simulink library "MinSegLibrary_M2V3"  (R2015a)
settings: Solver=ode45  StartTime=0.0  StopTime=10.0  RelTol=1e-3
libraries: arduinolib x4
settings Model: Creator=hurstj  LastModifiedBy=008399924
settings DebuggingCC: UnderspecifiedInitializationDetection=Classic  MergeDetectMultiDrivingBlocksExec=none  SolverPrmCheckMsg=warning  StateNameClashWarn=warning

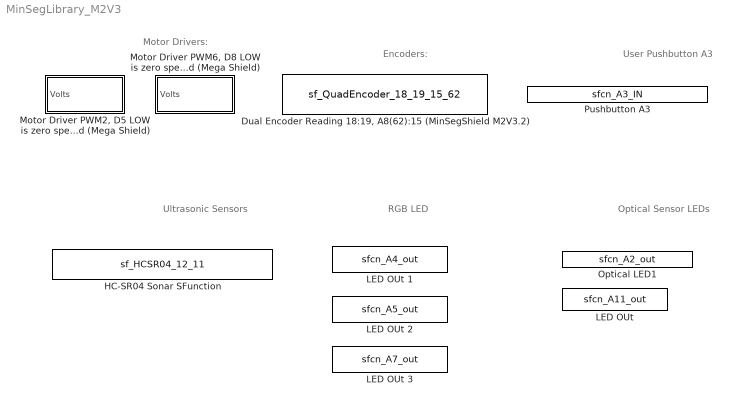
== system MinSegLibrary_M2V3 ==
  note: Motor Drivers:
  note: Ultrasonic Sensors
  note: Encoders:
  note: RGB LED
  note: User Pushbutton A3
  note: Optical Sensor LEDs
  "Dual Encoder Reading 18:19, A8(62):15 (MinSegShield M2V3.2) " : S-Function  InitFcn=try, set_param(gcb,'FunctionName','sf_QuadEncoder_18_19_15_62'), end  FunctionName=sf_QuadEncoder_18_19_15_62  Parameters=uint8([0 1]),uint8([18 62]),uint8([19 15])  SFunctionModules=sf_QuadEncoder_18_19_15_62_wrapper  mask(S-Function Builder){}
      mask init:
      | val = [[.9  0.75 0.75 1 1 .9 .9 1]',[1 1 0.75 0.75 .9 .9 1 .9]'];try , sys = get_param(gcb,'SfunBuilderFcnName');if isempty(sys), sys = get_param(gcb,'FunctionName'); end,catch, sys = get_param(gcb,'FunctionName'); end
      settings: CopyFcn=set_param(gcbh,'LinkStatus','none')  PreSaveFcn=try, set_param(gcb,'FunctionName','sf_QuadEncoder_18_19_15_62'), end  OpenFcn=sfunctionwizard(gcbh)
      mask Display: plot(val(:,1),val(:,2)),disp(sys), port_label('output',1,'pos1'), port_label('output',2,'pos2')
  HC-SR04 Sonar SFunction : S-Function  InitFcn=try, set_param(gcb,'FunctionName','sf_HCSR04_12_11'), end  FunctionName=sf_HCSR04_12_11  SFunctionModules=sf_HCSR04_12_11_wrapper  mask(S-Function Builder){}
      mask help: Simulink:masks:SFunctionBuilder_MD
      mask init: same as MinSegLibrary_M2V3/Dual Encoder Reading 18:19, A8(62):15 (MinSegShield M2V3.2) 
      settings: CopyFcn=set_param(gcbh,'LinkStatus','none')  PreSaveFcn=try, set_param(gcb,'FunctionName','sf_HCSR04_12_11'), end  OpenFcn=sfunctionwizard(gcbh)
      mask Display:
      | plot(val(:,1),val(:,2))
      | disp(sys)
      | port_label('output',1,'distance_cm')
  "LED OUt " : S-Function  InitFcn=try, set_param(gcb,'FunctionName','sfcn_A11_out'), end  FunctionName=sfcn_A11_out  Parameters=uint8(12)  SFunctionModules=sfcn_A11_out_wrapper  mask(S-Function Builder){}
      mask init: same as MinSegLibrary_M2V3/Dual Encoder Reading 18:19, A8(62):15 (MinSegShield M2V3.2) 
      settings: CopyFcn=set_param(gcbh,'LinkStatus','none')  PreSaveFcn=try, set_param(gcb,'FunctionName','sfcn_A11_out'), end  OpenFcn=sfunctionwizard(gcbh)
      mask Display: plot(val(:,1),val(:,2)),disp(sys), port_label('input',1,'in')
  LED OUt 1 : S-Function  InitFcn=try, set_param(gcb,'FunctionName','sfcn_A4_out'), end  FunctionName=sfcn_A4_out  Parameters=uint8(12)  SFunctionModules=sfcn_A4_out_wrapper  mask(S-Function Builder){}
      mask init: same as MinSegLibrary_M2V3/Dual Encoder Reading 18:19, A8(62):15 (MinSegShield M2V3.2) 
      settings: CopyFcn=set_param(gcbh,'LinkStatus','none')  PreSaveFcn=try, set_param(gcb,'FunctionName','sfcn_A4_out'), end  OpenFcn=sfunctionwizard(gcbh)
      mask Display: plot(val(:,1),val(:,2)),disp(sys), port_label('input',1,'in')
  LED OUt 2 : S-Function  InitFcn=try, set_param(gcb,'FunctionName','sfcn_A5_out'), end  FunctionName=sfcn_A5_out  Parameters=uint8(12)  SFunctionModules=sfcn_A5_out_wrapper  mask(S-Function Builder){}
      mask init: same as MinSegLibrary_M2V3/Dual Encoder Reading 18:19, A8(62):15 (MinSegShield M2V3.2) 
      settings: CopyFcn=set_param(gcbh,'LinkStatus','none')  PreSaveFcn=try, set_param(gcb,'FunctionName','sfcn_A5_out'), end  OpenFcn=sfunctionwizard(gcbh)
      mask Display: plot(val(:,1),val(:,2)),disp(sys), port_label('input',1,'in')
  LED OUt 3 : S-Function  InitFcn=try, set_param(gcb,'FunctionName','sfcn_A7_out'), end  FunctionName=sfcn_A7_out  Parameters=uint8(12)  SFunctionModules=sfcn_A7_out_wrapper  mask(S-Function Builder){}
      mask init: same as MinSegLibrary_M2V3/Dual Encoder Reading 18:19, A8(62):15 (MinSegShield M2V3.2) 
      settings: CopyFcn=set_param(gcbh,'LinkStatus','none')  PreSaveFcn=try, set_param(gcb,'FunctionName','sfcn_A7_out'), end  OpenFcn=sfunctionwizard(gcbh)
      mask Display: plot(val(:,1),val(:,2)),disp(sys), port_label('input',1,'in')
  "Motor Driver PWM2, D5 LOW is zero speed (Mega Shield)" : Subsystem
  "Motor Driver PWM6, D8 LOW is zero speed (Mega Shield)" : Subsystem
  Optical LED1 : S-Function  InitFcn=try, set_param(gcb,'FunctionName','sfcn_A2_out'), end  FunctionName=sfcn_A2_out  Parameters=uint8(12)  SFunctionModules=sfcn_A2_out_wrapper  mask(S-Function Builder){}
      mask init: same as MinSegLibrary_M2V3/Dual Encoder Reading 18:19, A8(62):15 (MinSegShield M2V3.2) 
      settings: CopyFcn=set_param(gcbh,'LinkStatus','none')  PreSaveFcn=try, set_param(gcb,'FunctionName','sfcn_A2_out'), end  OpenFcn=sfunctionwizard(gcbh)
      mask Display: plot(val(:,1),val(:,2)),disp(sys), port_label('input',1,'in')
  Pushbutton A3 : S-Function  InitFcn=try, set_param(gcb,'FunctionName','sfcn_A3_IN'), end  FunctionName=sfcn_A3_IN  SFunctionModules=sfcn_A3_IN_wrapper  mask(S-Function Builder){}
      mask help: Simulink:masks:SFunctionBuilder_MD
      mask init: same as MinSegLibrary_M2V3/Dual Encoder Reading 18:19, A8(62):15 (MinSegShield M2V3.2) 
      settings: CopyFcn=set_param(gcbh,'LinkStatus','none')  PreSaveFcn=try, set_param(gcb,'FunctionName','sfcn_A3_IN'), end  OpenFcn=sfunctionwizard(gcbh)
      mask Display: plot(val(:,1),val(:,2)),disp(sys), port_label('output',1,'push_button')

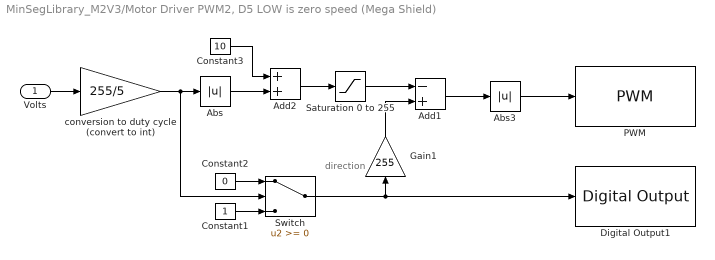
== system MinSegLibrary_M2V3/Motor Driver PWM2, D5 LOW is zero speed (Mega Shield) ==
  note: direction
  Volts : Inport
  Abs : Abs
  Abs3 : Abs
  Add1 : Sum  Inputs=-+
  Add2 : Sum
  Constant1 : Constant
  Constant2 : Constant  Value=0
  Constant3 : Constant  Value=10
  Digital Output1 : arduinolib/Digital Output  pinNumber=5
  Gain1 : Gain  Gain=255
  PWM : arduinolib/PWM  pinNumber=2
  Saturation 0 to 255 : Saturate  UpperLimit=255  LowerLimit=0
  Switch : Switch
  conversion to duty cycle (convert to int) : Gain  Gain=255/5  OutDataTypeStr=int16
  wires:
  Volts/1 -> conversion to duty cycle (convert to int)/1
  Switch/1 -> Digital Output1/1, Gain1/1
  Constant2/1 -> Switch/1
  Constant1/1 -> Switch/3
  Gain1/1 -> Add1/2
  Add1/1 -> Abs3/1
  conversion to duty cycle (convert to int)/1 -> Switch/2, Abs/1
  Saturation 0 to 255/1 -> Add1/1
  Abs3/1 -> PWM/1
  Constant3/1 -> Add2/1
  Abs/1 -> Add2/2
  Add2/1 -> Saturation 0 to 255/1

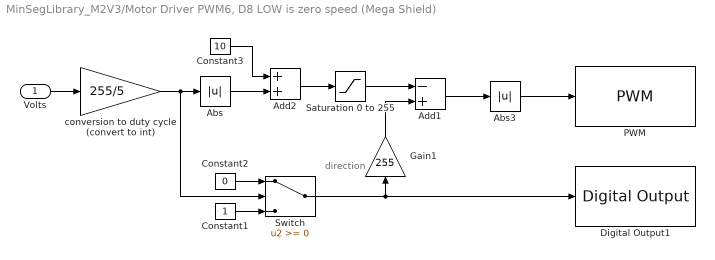
== system MinSegLibrary_M2V3/Motor Driver PWM6, D8 LOW is zero speed (Mega Shield) ==
  note: direction
  Volts : Inport
  Abs : Abs
  Abs3 : Abs
  Add1 : Sum  Inputs=-+
  Add2 : Sum
  Constant1 : Constant
  Constant2 : Constant  Value=0
  Constant3 : Constant  Value=10
  Digital Output1 : arduinolib/Digital Output  pinNumber=8
  Gain1 : Gain  Gain=255
  PWM : arduinolib/PWM  pinNumber=6
  Saturation 0 to 255 : Saturate  UpperLimit=255  LowerLimit=0
  Switch : Switch
  conversion to duty cycle (convert to int) : Gain  Gain=255/5  OutDataTypeStr=int16
  wires:
  Volts/1 -> conversion to duty cycle (convert to int)/1
  Switch/1 -> Digital Output1/1, Gain1/1
  Constant2/1 -> Switch/1
  Constant1/1 -> Switch/3
  Gain1/1 -> Add1/2
  Add1/1 -> Abs3/1
  conversion to duty cycle (convert to int)/1 -> Switch/2, Abs/1
  Saturation 0 to 255/1 -> Add1/1
  Abs3/1 -> PWM/1
  Constant3/1 -> Add2/1
  Abs/1 -> Add2/2
  Add2/1 -> Saturation 0 to 255/1
